simulink model "TST_StateflowHistoryJunction"  (Simulink 10.0)
settings: Solver=FixedStepDiscrete  StartTime=0.0  StopTime=10.0  FixedStep=0.02  RelTol=1e-3  EnableMultiTasking=on
settings Model: Creator=kharthforeign  LastModifiedBy=unknown
settings DataIOCC: LimitDataPoints=on  SignalLoggingSaveFormat=ModelDataLogs  SaveOutput=off  SignalLogging=off  SaveTime=off
settings OptimizationCC: BlockReduction=off  ConditionallyExecuteInputs=off  OptimizeBlockIOStorage=off  BufferReuse=off  GlobalBufferReuse=off  ExpressionFolding=off  ExpressionDepthLimit=2147483647  LocalBlockOutputs=off  InitFltsAndDblsToZero=on  OptimizeDataStoreBuffers=off  BusAssignmentInplaceUpdate=off
settings DebuggingCC: SolverPrmCheckMsg=warning  FcnCallInpInsideContextMsg=warning  StateNameClashWarn=warning
settings SFSimCC: SimParseCustomCode=off
settings GRTTargetCC: GeneratePreprocessorConditionals=Disable all
settings ConfigComp: CovExternalEMLEnable=off

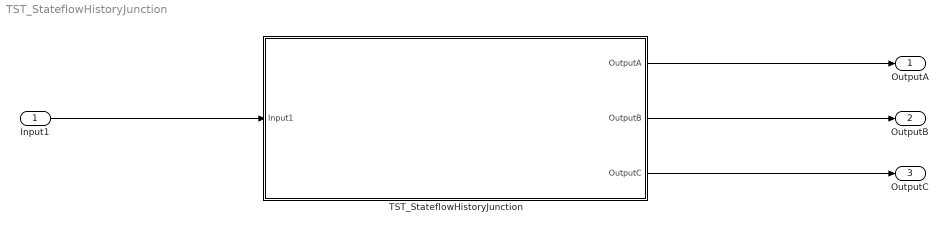
== system TST_StateflowHistoryJunction ==
  Input1 : Inport  OutDataTypeStr=uint32  BusOutputAsStruct=on
  TST_StateflowHistoryJunction : Subsystem  TreatAsAtomicUnit=on
  OutputA : Outport  OutDataTypeStr=double  PortDimensions=1
  OutputB : Outport  Port=2  OutDataTypeStr=double  PortDimensions=1
  OutputC : Outport  Port=3  OutDataTypeStr=double  PortDimensions=1
  wires:
  Input1/1 -> TST_StateflowHistoryJunction/1(Input1)
  TST_StateflowHistoryJunction/1(OutputA) -> OutputA/1
  TST_StateflowHistoryJunction/2(OutputB) -> OutputB/1
  TST_StateflowHistoryJunction/3(OutputC) -> OutputC/1

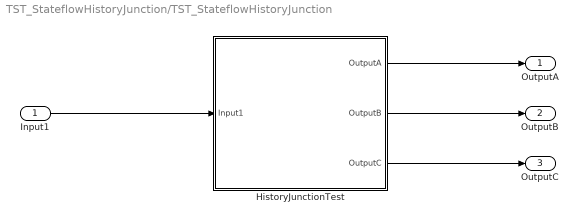
== system TST_StateflowHistoryJunction/TST_StateflowHistoryJunction ==
  Input1 : Inport  OutDataTypeStr=uint32  BusOutputAsStruct=on
  HistoryJunctionTest : Stateflow chart  TreatAsAtomicUnit=on
  OutputA : Outport  OutDataTypeStr=double  PortDimensions=1
  OutputB : Outport  Port=2  OutDataTypeStr=double  PortDimensions=1
  OutputC : Outport  Port=3  OutDataTypeStr=double  PortDimensions=1
  wires:
  HistoryJunctionTest/1(OutputA) -> OutputA/1
  HistoryJunctionTest/2(OutputB) -> OutputB/1
  HistoryJunctionTest/3(OutputC) -> OutputC/1
  Input1/1 -> HistoryJunctionTest/1(Input1)

== stateflow chart TST_StateflowHistoryJunction/HistoryJunctionTest ==
  state TopStateWithHistory
    entry:
    Local = uint32(10);
    exit:
    Local = uint32(20);
    (history)
    state SubState2A
      entry:
      OutputA = uint32(10);
      exit:
      OutputA = uint32(20);
    state SubState2B
      entry:
      OutputB = uint32(10);
      exit:
      OutputB = uint32(20);
    state SubState2C
      entry:
      OutputC = uint32(10);
      exit:
      OutputC = uint32(20);
    (default) -> SubState2A
    SubState2A -> SubState2B : [A && B]
    SubState2C -> SubState2A [order 2] : [C && A]
    SubState2B -> SubState2C [order 2] : [B && C]
  state TopStateNoHistory
    entry:
    Local = uint32(1);
    exit:
    Local = uint32(2);
    state SubState1C
      entry:
      OutputC = uint32(1);
      exit:
      OutputC = uint32(2);
    state SubState1A
      entry:
      OutputA = uint32(1);
      exit:
      OutputA = uint32(2);
    state SubState1B
      entry:
      OutputB = uint32(1);
      exit:
      OutputB = uint32(2);
    (default) -> SubState1A
    SubState1A -> SubState1B : [A && B]
    SubState1C -> SubState1A [order 2] : [C && A]
    SubState1B -> SubState1C [order 2] : [B && C]
  TopStateNoHistory -> SubState2A [order 1] : [A &&  ~B]
  TopStateWithHistory -> SubState1A [order 1] : [A && ~B]
  (default) -> TopStateNoHistory
  TopStateNoHistory -> TopStateWithHistory [order 2] : [A]
  TopStateWithHistory -> TopStateNoHistory [order 2] : [A]
  SubState2B -> SubState1B [order 1] : [B]
  SubState1B -> SubState2B [order 1] : [B]
  SubState1C -> TopStateWithHistory [order 1] : [C]
  SubState2C -> TopStateNoHistory [order 1] : [C]
  data: Input1 input uint32; OutputA output double =1; OutputB output double =2; OutputC output double =3; Local local uint32 =0; A local boolean; B local boolean; C local boolean
